simulink model "model_negation_operative_temp"  (R2019b)
settings: Solver=FixedStepAuto  StartTime=0.0  StopTime=40  FixedStep=0.1  RelTol=1e-3
values from neighbouring files (symbols this model uses):
  nb_rooms = 4    [full_test.m]
  nb_second_in_timeunit = 60*5    (= 300)    [full_test.m]
  timeunit_in_a_day = 2*6*24    (= 288)    [full_test.m]
undefined symbols (not defined in the file or in its folder): air_mass_kg_rooms, Area_boiler, area_outdoor_rooms, Area_radiators, area_rooms_ground, area_walls_between_rooms, C_air, C_water, Energy_used_by_air_conditioner_for_1_timeunit_in_Watts_vector, Energy_used_by_air_mixer_for_1_timeunit_in_Watts, Energy_used_by_boiler_for_1_timeunit_in_Watts, initial_relative_humidity, initial_temp_water_in_boilers, initial_temperature_rooms, initial_temperature_water_in_radiator, k_boiler_border, k_radiators, k_wall_outdoor_rooms, k_walls_between_rooms, mass_water_radiator, matrix_AC_rooms_locations, matrix_boiler_radiator_connection, matrix_boiler_rooms_locations, matrix_radiator_rooms_locations, nb_air_cons, nb_boilers, nb_humans, nb_radiators, outdoor_max_temp_A, outdoor_max_temp_B, outdoor_min_temp_A, outdoor_min_temp_B, tau_boiler, thickness_boiler, thickness_outdoor_rooms, thickness_radiator_pipes, thickness_walls_between_rooms, Volume_radiators, Volume_rooms, water_weight_in_boiler, watt_generation_of_employe
libraries: dspmtrx3 x15, dspstat3 x3, simulink x2
(part 2 of 2)

== system model_negation_operative_temp/Physical model/Wall heat Exchange module/Value heat exchange within building ==
  "T_rooms " : Inport
  Constant : Constant  Value=diag(ones(nb_rooms,1))
  Gain3 : Gain  Gain=area_walls_between_rooms
  Gain4 : Gain  Gain=k_walls_between_rooms
  Gain8 : Gain  Gain=ones(nb_rooms,nb_rooms)./thickness_walls_between_rooms
  MATRIX WITH ROOM TEMPERATURE DIFFERENCE The area matrix after handles the case of non-adjacent rooms : dspmtrx3/Array-Vector Multiply  mode=Mute  saveAsFlag=0  Dimension=2  V_Source=Input port  V_VectFromMask=[0.5 0.25]  roundingMode=Floor  overflowMode=off  firstCoeffSignedness=Auto  firstCoeffDataTypeStr=Inherit: Same word length as input  firstCoeffMin=[]  firstCoeffMax=[]  firstCoeffLastDataTypeStr=Inherit: Same word length as input  prodOutputSignedness=Auto  accumSignedness=Auto  outputSignedness=Auto  outputDataTypeStr=Inherit: Same as product output  outputMin=[]  outputMax=[]  outputLastDataTypeStr=Inherit: Same as product output
      settings: SourceProductName=DSP System Toolbox  SourceProductBaseCode=DS
  Sum of Elements : Sum  Inputs=+  CollapseMode=Specified dimension  CollapseDim=2
  Q_in_building_to_rooms : Outport
  wires:
  Gain4/1 -> Gain8/1
  Gain3/1 -> Gain4/1
  MATRIX WITH ROOM TEMPERATURE DIFFERENCE The area matrix after handles the case of non-adjacent rooms/1 -> Gain3/1
  Gain8/1 -> Sum of Elements/1
  Sum of Elements/1 -> Q_in_building_to_rooms/1
  Constant/1 -> MATRIX WITH ROOM TEMPERATURE DIFFERENCE The area matrix after handles the case of non-adjacent rooms/1
  "T_rooms "/1 -> MATRIX WITH ROOM TEMPERATURE DIFFERENCE The area matrix after handles the case of non-adjacent rooms/2

== matlab function model_negation_operative_temp/specification verification module/gt ss epsilon = 1/MATLAB Function operative temp ==
  data: s input; y output
function y = fcn(s)
	
    y = zeros(size(s,1),1);

    function yy = fbis(ee)
        left = 23.5-ee; 
        right = ee-26.5;    
        yy = max(left,right); % or
    end

    for i=1:size(s,1)
        ss = s(i);
        [a b] =  fminbnd(@fbis,ss-1,ss+1);  
        y(i)=a-ss;
    end
    
end

== matlab function model_negation_operative_temp/specification verification module/gt ss epsilon = 0.5/MATLAB Function operative temp ==
  data: s input; y output
function y = fcn(s)
	
    y = zeros(size(s,1),1);

    function yy = fbis(ee)
        left = 23.5-ee; 
        right = ee-26.5;    
        yy = max(left,right); % or
    end

    for i=1:size(s,1)
        ss = s(i);
        [a b] =  fminbnd(@fbis,ss-0.5,ss+0.5);  
        y(i)=a-ss;
    end
    
end
